simulink model "q1"  (R2020a)
settings: Solver=FixedStepDiscrete  StartTime=0.0  StopTime=127  FixedStep=1  RelTol=1e-3
settings Model: Creator=ACER  LastModifiedBy=ACER

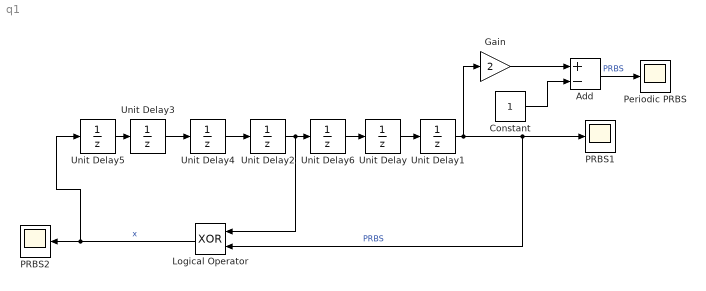
== system q1 ==
  Add : Sum  Inputs=+-
  Constant : Constant
  Gain : Gain  Gain=2
  Logical Operator : Logic  Operator=XOR  AllPortsSameDT=off  OutDataTypeStr=boolean
  PRBS1 : Scope
  PRBS2 : Scope
  Periodic PRBS : Scope
  Unit Delay{,1,4..6} (5 alike) : UnitDelay  InitialCondition=1  SampleTime=-1  HasFrameUpgradeWarning=on
  Unit Delay2 : UnitDelay  SampleTime=-1  HasFrameUpgradeWarning=on
  Unit Delay3 : UnitDelay  SampleTime=-1  HasFrameUpgradeWarning=on
  wires:
  Logical Operator/1 -> Unit Delay5/1, PRBS2/1  "x"
  Unit Delay/1 -> Unit Delay1/1
  Unit Delay2/1 -> Logical Operator/1, Unit Delay6/1
  Unit Delay1/1 -> Gain/1, Logical Operator/2, PRBS1/1  "PRBS"
  Gain/1 -> Add/1
  Add/1 -> Periodic PRBS/1  "PRBS"
  Constant/1 -> Add/2
  Unit Delay3/1 -> Unit Delay4/1
  Unit Delay4/1 -> Unit Delay2/1
  Unit Delay5/1 -> Unit Delay3/1
  Unit Delay6/1 -> Unit Delay/1
